simulink model "motor_control"  (R2024b)
settings: Solver=VariableStepAuto  StartTime=0.0  StopTime=3.0  RelTol=1e-3
model workspace (MAT data in the model file):
  K = 12
values from neighbouring files (symbols this model uses):
  k = 1.9    [Comparemotorsim.m]    (also in Runcontrolsim.m; Runmotorsim.m = 2.2)
  Kp = 10    [Runcontrolsim.m]
  sigma = 18    [Comparemotorsim.m]    (also in Runcontrolsim.m; Runmotorsim.m = 2)
libraries: simulink x1
settings Model: Creator=jesus  LastModifiedBy=jesus

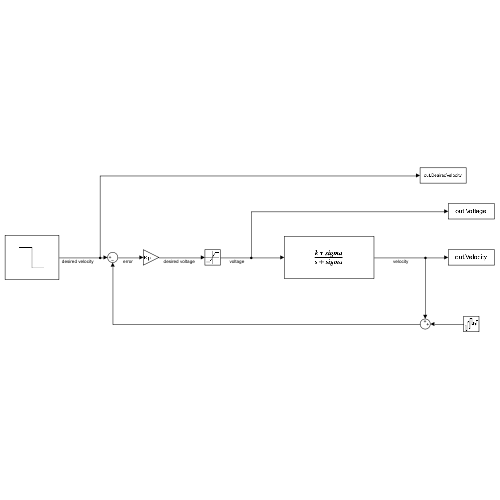
[thumbnail: Simulink's stored preview of the top-level diagram]
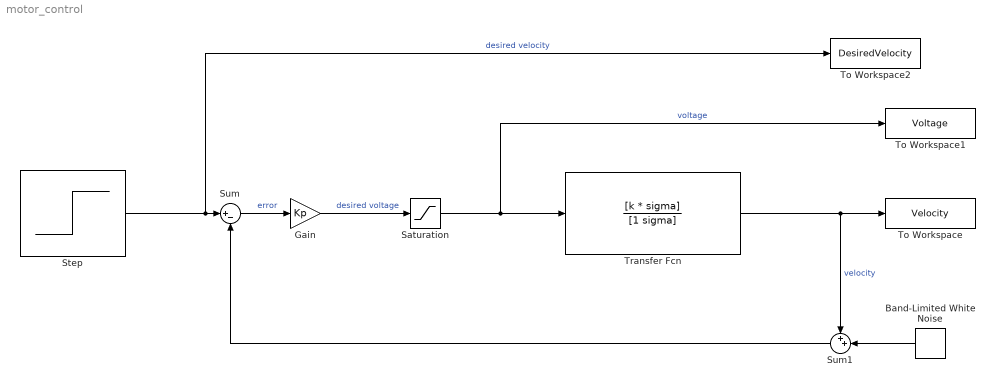
== system motor_control ==
  Band-Limited White Noise : simulink/Sources/Band-Limited White Noise  Cov=[0.0001]  Ts=0.01  seed=[23341]
  Gain : Gain  Gain=Kp
  Saturation : Saturate  UpperLimit=7.5  LowerLimit=-7.5
  Step : Step  Time=0  After=-6.28  SampleTime=0
  Sum : Sum  Inputs=|+-
  Sum1 : Sum  Inputs=++|
  To Workspace : ToWorkspace  VariableName=Velocity  SaveFormat=Timeseries  SampleTime=-1
  To Workspace1 : ToWorkspace  VariableName=Voltage  SaveFormat=Timeseries  SampleTime=-1
  To Workspace2 : ToWorkspace  VariableName=DesiredVelocity  SaveFormat=Timeseries  SampleTime=-1
  Transfer Fcn : TransferFcn  Numerator=[k * sigma]  Denominator=[1 sigma]
  wires:
  Transfer Fcn/1 -> Sum1/1, To Workspace/1  "velocity"
  Step/1 -> To Workspace2/1, Sum/1  "desired velocity"
  Sum/1 -> Gain/1  "error"
  Gain/1 -> Saturation/1  "desired voltage"
  Saturation/1 -> To Workspace1/1, Transfer Fcn/1  "voltage"
  Sum1/1 -> Sum/2
  Band-Limited White Noise/1 -> Sum1/2
